simulink model "model_sim_2023b"  (R2025a)
settings: Solver=VariableStepAuto  StartTime=0.0  StopTime=10  MaxStep=1e-3  RelTol=1e-3
values from neighbouring files (symbols this model uses):
  dead_zone_width = double(mod.DEAD_ZONE_WIDTH)    [simulation__data.m]
  dir_coeff = double(mod.direct_conv_fun_coeff)    [simulation__data.m]
  inv_coeff = double(mod.inverse_conv_fun_coeff)    [simulation__data.m]
  max_PWM = double(mod.MAX_PWM)    [simulation__data.m]
  pulse_zero = pulse_min    (= 10)    [simulation__data.m]
  step_0_pulse_1 = 1    [simulation__data.m]
  step_value = 20    [simulation__data.m]
  T_sampling = double(mod.SAMPLING_PERIOD)    [simulation__data.m]
  x0 = 50    [simulation__data.m]
undefined symbols (not defined in the file or in its folder): DG_coeff, NG_coeff
settings Model: Creator=feder  LastModifiedBy=Federico Romairone

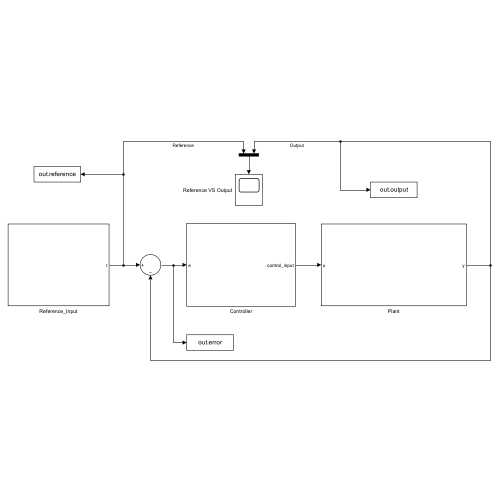
[thumbnail: Simulink's stored preview of the top-level diagram]
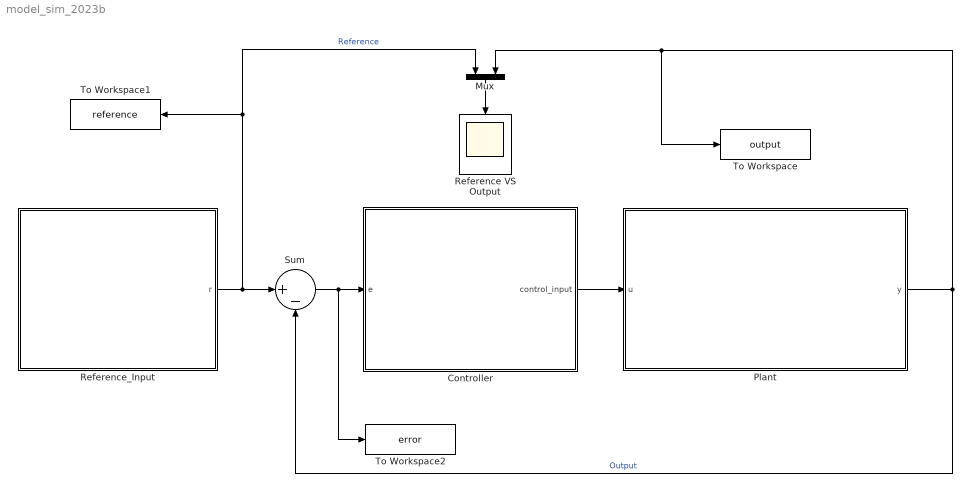
== system model_sim_2023b ==
  Controller : Subsystem
  Mux : Mux  Inputs=2
  Plant : Subsystem
  Reference VS Output : Scope
      settings: ActiveDisplayYMinimum=0.50345417341726884  ActiveDisplayYMaximum=1.2057933689055544
  Reference_Input : Subsystem
  Sum : Sum  Inputs=|+-
  To Workspace : ToWorkspace  VariableName=output  SaveFormat=Timeseries  SampleTime=-1
  To Workspace1 : ToWorkspace  VariableName=reference  SaveFormat=Timeseries  SampleTime=-1
  To Workspace2 : ToWorkspace  VariableName=error  SaveFormat=Timeseries  SampleTime=-1
  wires:
  Plant/1(y) -> Sum/2, To Workspace/1, Mux/2  "Output"
  Sum/1 -> To Workspace2/1, Controller/1(e)
  Controller/1(control_input) -> Plant/1(u)
  Mux/1 -> Reference VS Output/1
  Reference_Input/1(r) -> To Workspace1/1, Mux/1, Sum/1  "Reference"

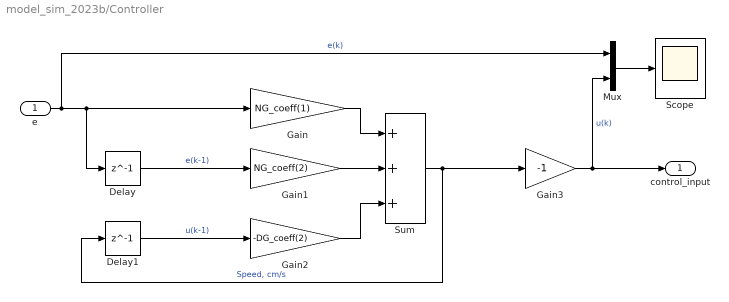
== system model_sim_2023b/Controller ==
  e : Inport
  Delay : Delay  DelayLength=1  InitialCondition=0  SampleTime=T_sampling
  Delay1 : Delay  DelayLength=1  InitialCondition=0  SampleTime=T_sampling
  Gain : Gain  Gain=NG_coeff(1)
  Gain1 : Gain  Gain=NG_coeff(2)
  Gain2 : Gain  Gain=-DG_coeff(2)
  Gain3 : Gain  Gain=-1
  Mux : Mux  Inputs=2
  Scope : Scope
      settings: ActiveDisplayYMinimum=-23.638854557377861  ActiveDisplayYMaximum=0.35923089484270676  DataLoggingVariableName=ScopeData2
  Sum : Sum  Inputs=+++
  control_input : Outport
  wires:
  e/1 -> Mux/1, Delay/1, Gain/1  "e(k)"
  Sum/1 -> Gain3/1, Delay1/1  "Speed, cm/s"
  Gain3/1 -> Mux/2, control_input/1  "u(k)"
  Delay/1 -> Gain1/1  "e(k-1)"
  Delay1/1 -> Gain2/1  "u(k-1)"
  Gain/1 -> Sum/1
  Gain1/1 -> Sum/2
  Gain2/1 -> Sum/3
  Mux/1 -> Scope/1

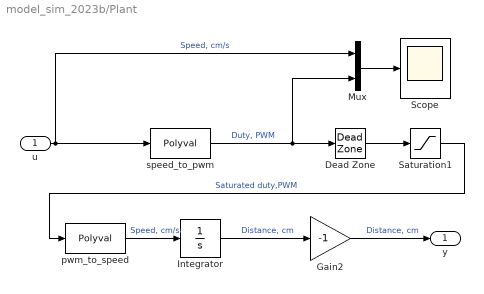
== system model_sim_2023b/Plant ==
  u : Inport
  Dead Zone : DeadZone  LowerValue=-dead_zone_width  UpperValue=dead_zone_width
  Gain2 : Gain  Gain=-1
  Integrator : Integrator  InitialCondition=-x0
  Mux : Mux  Inputs=2
  Saturation1 : Saturate  UpperLimit=max_PWM  LowerLimit=-max_PWM
  Scope : Scope
      settings: ActiveDisplayYMinimum=-841.36472677049653  ActiveDisplayYMaximum=5.5331943573754643  DataLoggingVariableName=ScopeData7
  pwm_to_speed : Polyval  Coefs=inv_coeff
  speed_to_pwm : Polyval  Coefs=dir_coeff
  y : Outport
  wires:
  Integrator/1 -> Gain2/1  "Distance, cm"
  Gain2/1 -> y/1  "Distance, cm"
  speed_to_pwm/1 -> Dead Zone/1, Mux/2  "Duty, PWM"
  u/1 -> speed_to_pwm/1, Mux/1  "Speed, cm/s"
  Dead Zone/1 -> Saturation1/1
  Mux/1 -> Scope/1
  pwm_to_speed/1 -> Integrator/1  "Speed, cm/s"
  Saturation1/1 -> pwm_to_speed/1  "Saturated duty,PWM"

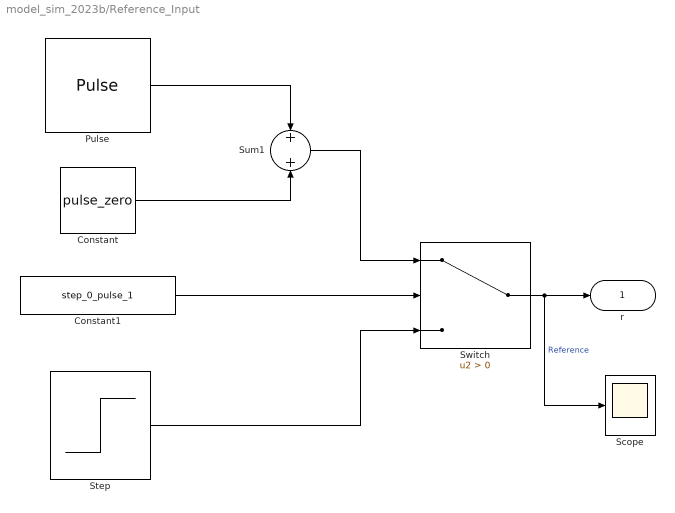
== system model_sim_2023b/Reference_Input ==
  Constant : Constant  Value=pulse_zero
  Constant1 : Constant  Value=step_0_pulse_1
  Pulse : DiscretePulseGenerator  PulseType=Time based  Amplitude=step_value  Period=4  PulseWidth=50
  Scope : Scope
      settings: ActiveDisplayYMinimum=0.9  ActiveDisplayYMaximum=1.1  DataLoggingVariableName=ScopeData6
  Step : Step  Time=0  After=step_value  SampleTime=0
  Sum1 : Sum
  Switch : Switch  Criteria=u2 > Threshold  SaturateOnIntegerOverflow=off  InputSameDT=off
  r : Outport
  wires:
  Pulse/1 -> Sum1/1
  Constant/1 -> Sum1/2
  Constant1/1 -> Switch/2
  Sum1/1 -> Switch/1
  Step/1 -> Switch/3
  Switch/1 -> r/1, Scope/1  "Reference"
